simulink model "s_torce2"  (Simulink 4.00)
settings: Solver=ode45  SolverMode=SingleTasking  StartTime=0.0  StopTime=50  FixedStep=0.1  MaxStep=0.1  RelTol=1e-3  AbsTol=1e-6
values from neighbouring files (symbols this model uses):
  A1 = 2    [torce11.m]    (also in torcell.mat; waag11.mat)
  A12 = 0.1    [torce11.m]    (also in torcell.mat; waag11.mat)
  A2 = 2    [torce11.m]    (also in torcell.mat; waag11.mat)
  g = 9.8    [ident21.mat]    (also in torce11.m = 9.81; torcell.mat = 9.81; waag11.m = 9.81; waag11.mat = 9.81)
  kd = 15    [torce11.m]    (also in torcell.mat = 161.02296887; waag11.m = 10; waag11.mat = 9.39541279526; waage2.m = ',num2str(kd),' ;']))
  ki = 1    [ncd_estim1.m]    (also in ncd_estim_1.mat = 1.82974576844; ncd_kalm1.m; ncd_kalm2.m; ncd_kalm_1.mat = 1.97821802246)
  kp = 5    [torce11.m]    (also in torcell.mat = -9.12500428484; waag11.m = 100; waag11.mat = 270.25934718; waage2.m = 100)
  N = 20    [torce11.m]    (also in torcell.mat = 20.6513238556; waag11.m; waag11.mat; waage2.m)
  Qz_max = 4    [torce11.m]    (also in torcell.mat; waag11.mat)
  Qz_min = 0    [torce11.m]    (also in torcell.mat; waag11.mat)
libraries: simulink_extras x1
settings Model: LastModifiedBy=Administrator  SaveTime=off  SaveOutput=off  LimitDataPoints=off  BlockReductionOpt=off

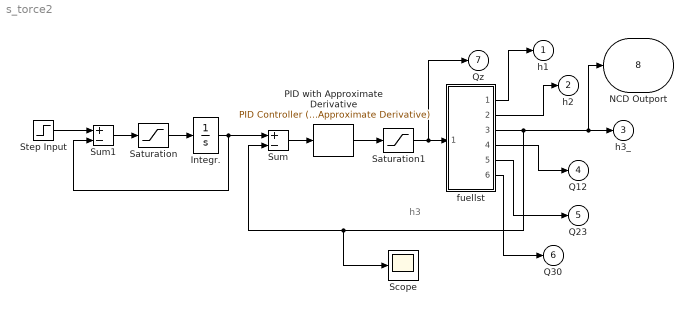
== system s_torce2 ==
  note: h3
  "Integr. " : Integrator  ExternalReset=none  InitialConditionSource=internal  InitialCondition=0  LimitOutput=off  UpperSaturationLimit=inf  LowerSaturationLimit=-inf  ShowSaturationPort=off  ShowStatePort=off  AbsoluteTolerance=auto
  PID with Approximate Derivative : simulink_extras/Additional Linear/PID Controller (with Approximate Derivative)  P=kp  I=ki  D=kd  N=N
  Saturation : Saturate  UpperLimit=0.1  LowerLimit=-0.1  LinearizeAsGain=on
  Saturation1 : Saturate  UpperLimit=Qz_max  LowerLimit=Qz_min  LinearizeAsGain=on
  Scope : Scope
      settings: TickLabels=on  TimeRange=50.000000  YMin=-3.000000  YMax=3.000000  SaveToWorkspace=off  SaveName=ScopeData  DataFormat=Array  LimitDataPoints=on  MaxDataPoints=5000
  Step Input : Step  Time=1  Before=0  After=1  SampleTime=0
  Sum : Sum  Inputs=+-  SaturateOnIntegerOverflow=on
  Sum1 : Sum  Inputs=+-  SaturateOnIntegerOverflow=on
  "fuellst " : Subsystem
      settings: RTWFcnNameOpts=Auto  RTWFileNameOpts=Auto
  h1 : Outport  Port=1
  h2 : Outport  Port=2
  h3_ : Outport  Port=3
  Q12 : Outport  Port=4
  Q23 : Outport  Port=5
  Q30 : Outport  Port=6
  Qz : Outport  Port=7
  NCD Outport : Outport  Port=8  InitialOutput=0
      settings: OpenFcn=optblock
      mask Type: NCD Outport
      mask Display:
      | plot([0:10],[-.5 1.5 .6 1.3 .8 1.1 .95 1.02 .99 1 1]);
      | disp('\n\n NCD\n OutPort 8');
  wires:
  Saturation1/1 -> Qz/1, "fuellst "/1(in_1)
  PID with Approximate Derivative/1 -> Saturation1/1
  "Integr. "/1 -> Sum1/2, Sum/1
  Step Input/1 -> Sum1/1
  Sum1/1 -> Saturation/1
  Saturation/1 -> "Integr. "/1
  "fuellst "/3(out_5) -> Scope/1, Sum/2, h3_/1, NCD Outport/1
  "fuellst "/6(out_6) -> Q30/1
  "fuellst "/5(out_4) -> Q23/1
  "fuellst "/4(out_2) -> Q12/1
  "fuellst "/2(out_3) -> h2/1
  "fuellst "/1(out_1) -> h1/1
  Sum/1 -> PID with Approximate Derivative/1

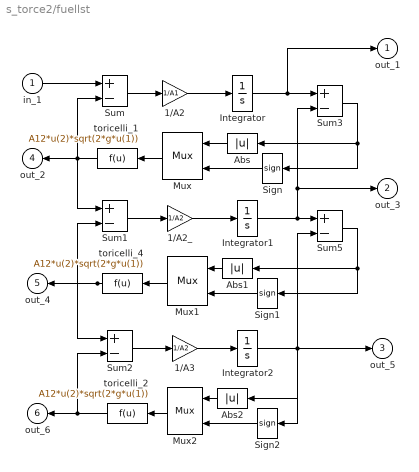
== system s_torce2/fuellst  ==
  in_1 : Inport  Port=1
  1/A2 : Gain  Gain=1/A1  Multiplication=Element-wise(K.*u)  SaturateOnIntegerOverflow=on
  1/A2_ : Gain  Gain=1/A2  Multiplication=Element-wise(K.*u)  SaturateOnIntegerOverflow=on
  1/A3 : Gain  Gain=1/A2  Multiplication=Element-wise(K.*u)  SaturateOnIntegerOverflow=on
  Abs : Abs  Orientation=left  SaturateOnIntegerOverflow=on
  Abs1 : Abs  Orientation=left  SaturateOnIntegerOverflow=on
  Abs2 : Abs  Orientation=left  SaturateOnIntegerOverflow=on
  Integrator : Integrator  ExternalReset=none  InitialConditionSource=internal  InitialCondition=0  LimitOutput=off  UpperSaturationLimit=inf  LowerSaturationLimit=-inf  ShowSaturationPort=off  ShowStatePort=off  AbsoluteTolerance=auto
  Integrator1 : Integrator  ExternalReset=none  InitialConditionSource=internal  InitialCondition=0  LimitOutput=off  UpperSaturationLimit=inf  LowerSaturationLimit=-inf  ShowSaturationPort=off  ShowStatePort=off  AbsoluteTolerance=auto
  Integrator2 : Integrator  ExternalReset=none  InitialConditionSource=internal  InitialCondition=0  LimitOutput=off  UpperSaturationLimit=inf  LowerSaturationLimit=-inf  ShowSaturationPort=off  ShowStatePort=off  AbsoluteTolerance=auto
  Mux : Mux  Orientation=left  Inputs=2
      settings: DisplayOption=none
  Mux1 : Mux  Orientation=left  Inputs=2
      settings: DisplayOption=none
  Mux2 : Mux  Orientation=left  Inputs=2
      settings: DisplayOption=none
  Sign : Signum  Orientation=left
  Sign1 : Signum  Orientation=left
  Sign2 : Signum  Orientation=left
  Sum{,1..3,5} (5 alike) : Sum  Inputs=+-  SaturateOnIntegerOverflow=on
  toricelli_1 : Fcn  Orientation=left  Expr=A12*u(2)*sqrt(2*g*u(1))
  toricelli_2 : Fcn  Orientation=left  Expr=A12*u(2)*sqrt(2*g*u(1))
  toricelli_4 : Fcn  Orientation=left  Expr=A12*u(2)*sqrt(2*g*u(1))
  out_1 : Outport  Port=1
  out_3 : Outport  Port=2
  out_5 : Outport  Port=3
  out_2 : Outport  Orientation=left  Port=4
  out_4 : Outport  Orientation=left  Port=5
  out_6 : Outport  Orientation=left  Port=6
  wires:
  in_1/1 -> Sum/1
  toricelli_2/1 -> Sum2/2, out_6/1
  Sign2/1 -> Mux2/2
  Mux2/1 -> toricelli_2/1
  Abs2/1 -> Mux2/1
  toricelli_4/1 -> Sum2/1, Sum1/2, out_4/1
  Abs1/1 -> Mux1/1
  Sum5/1 -> Sign1/1, Abs1/1
  Sign1/1 -> Mux1/2
  Mux1/1 -> toricelli_4/1
  Sign/1 -> Mux/2
  Mux/1 -> toricelli_1/1
  Abs/1 -> Mux/1
  Sum3/1 -> Sign/1, Abs/1
  toricelli_1/1 -> Sum1/1, Sum/2, out_2/1
  Integrator2/1 -> Sign2/1, Abs2/1, Sum5/2, out_5/1
  Integrator/1 -> Sum3/1, out_1/1
  1/A3/1 -> Integrator2/1
  1/A2_/1 -> Integrator1/1
  1/A2/1 -> Integrator/1
  Sum2/1 -> 1/A3/1
  Sum1/1 -> 1/A2_/1
  Sum/1 -> 1/A2/1
  Integrator1/1 -> Sum5/1, Sum3/2, out_3/1
